simulink model "soc_WLAN_fpga"  (R2024b)
settings: Solver=FixedStepDiscrete  StartTime=0.0  StopTime=stopTime  RelTol=1e-3
PreLoadFcn:
  | addpath(fullfile(matlabroot,'toolbox','whdl','whdlexamples','whdlexamples'));
InitFcn:
  | addpath(fullfile(matlabroot,'toolbox','whdl','whdlexamples','whdlexamples'));
model workspace (MAT data in the model file):
  socvcb : containers.Map (value not decoded)
undefined symbols (not defined in the file): Add, bitRatePerOfdmSym, chanBW, coe, cpLen, dataUpsampleFactor, DelayValMaxNsdMinusLastPilotSc, DescramblerInitialSeed, designMultirateFIR, fftLen, filterLatency, filterUpsampleFactor, Fs, Hd, HT_MFMCS0, HT_MFMCS1, HT_MFMCS2, HT_MFMCS3, HT_MFMCS4, HT_MFMCS5, HT_MFMCS6, HT_MFMCS7, HTUnUsedScInd, inputSamplingRate, interp_coeff, maxPilotRefCounterVale, maxPilotsRef, maxPilotsRefNonHT, Ncol_HT, Ncol_NonHT, noDataSubCarriers, Non_HTMCS0, Non_HTMCS1, Non_HTMCS2, Non_HTMCS3, Non_HTMCS4, Non_HTMCS5, Non_HTMCS6, Non_HTMCS7, Nrow_HT, Nrow_NonHT, numDSC_HT, numDSC_HT_vhtSigB, numDSC_NonHT, numDscHT, numDscNonHT, numOfBitsPerOFDMSym, numOfDataBitsPerOFDMSym, numPilots, numScHT, numSCS_HT, numSCS_NonHT, pnSeq, QAM, rxDownsampleFactor, secondPIdx_HT, secondPIdx_NonHT, Shift, VHTMCS0, VHTMCS1 ... (+7)
libraries: hdlsllib x267, simulink x210, dspsigops x22, whdlutilities x10, whdlmod x9, dsphdlfiltering2 x5, dsphdlmathfun2 x4, whdledac x3, hwlogicconnlib x2, commhdlcrc x2, dsphdlsigops2 x2
(part 4 of 14)

== system soc_WLAN_fpga/WLAN/WLAN HDL/WLAN_Tx_Rx/WLAN_Rx/WLANHDLReceiver/HT_VHTChannelEstAndEqualize/ChannelEqualizer ==
  note: Delay by 1 OFDM Symbol time
  dataIn : Inport
  validIn : Inport  Port=2
  chanEst : Inport  Port=3
  chanEstVal : Inport  Port=4
  chanEstLen : Inport  Port=5
  syncStart : Inport  Port=6
  symbNum : Inport  Port=7
  Delay1 : Delay  DelayLength=1
  Delay11 : Delay  DelayLength=1
  Delay2 : Delay  DelayLength=1
  Delay3 : Delay  DelayLength=80
  Delay4 : Delay  DelayLength=80
  Delay{5..6,8..9} (4 alike) : Delay
  HDL Counter : hdlsllib/Sources/HDL Counter  CountType=Count limited  CountInit=0  CountStep=1  CountMax=numSCS_HT-1  CountFromType=Initial value  CountFrom=0  CountResetPort=on  CountLoadPort=off  CountEnbPort=on  CountDirPort=off  CountHitOutputPort=off  CountDataType=Unsigned  CountWordLen=8  CountFracLen=0  CountSampTime=1
  HDL Counter1 : hdlsllib/Sources/HDL Counter  CountType=Count limited  CountInit=0  CountStep=1  CountMax=numSCS_HT-1  CountFromType=Initial value  CountFrom=0  CountResetPort=on  CountLoadPort=off  CountEnbPort=on  CountDirPort=off  CountHitOutputPort=off  CountDataType=Unsigned  CountWordLen=8  CountFracLen=0  CountSampTime=1
  OFDM Equalizer : whdlmod/OFDM Equalizer  EqualizationMethod=ZF  MaxLenChEstiPerSym=numSCS_HT  resetPort=on
  Simple Dual Port RAM1 : hdlsllib/HDL RAMs/Simple Dual Port RAM  ram_size=8
  validForEqualization : Subsystem
  dataOut : Outport
  validOut : Outport  Port=2
  wires:
  validForEqualization/1(hValid) -> HDL Counter1/2
  HDL Counter/1 -> Simple Dual Port RAM1/2
  validIn/1 -> validForEqualization/1(validIn)
  Delay11/1 -> Simple Dual Port RAM1/4
  HDL Counter1/1 -> Delay11/1
  Delay9/1 -> OFDM Equalizer/1
  Delay3/1 -> Delay1/1
  Delay8/1 -> OFDM Equalizer/4
  Delay6/1 -> OFDM Equalizer/5
  validForEqualization/3(loadH) -> Delay6/1
  Simple Dual Port RAM1/1 -> OFDM Equalizer/2
  Delay5/1 -> OFDM Equalizer/3
  dataIn/1 -> Delay9/1
  symbNum/1 -> validForEqualization/2(symbNum)
  Delay4/1 -> Delay2/1
  chanEstVal/1 -> Delay4/1
  chanEstLen/1 -> Delay8/1
  validForEqualization/2(DataValid) -> Delay5/1
  chanEst/1 -> Delay3/1
  OFDM Equalizer/2 -> validOut/1
  OFDM Equalizer/1 -> dataOut/1
  syncStart/1 -> HDL Counter1/1, validForEqualization/3(rst), OFDM Equalizer/6, HDL Counter/1
  Delay1/1 -> Simple Dual Port RAM1/1
  Delay2/1 -> Simple Dual Port RAM1/3, HDL Counter/2

== system soc_WLAN_fpga/WLAN/WLAN HDL/WLAN_Tx_Rx/WLAN_Rx/WLANHDLReceiver/HT_VHTChannelEstAndEqualize/ChannelEstimator ==
  note: Selecting 9th symbol i.e., HT/VHT LTF after OFDM demod
  note: Sending chan est as 1 when valid is low to channel equalizer
  dataIn : Inport
  validIn : Inport  Port=2
  syncStart : Inport  Port=3
  symbNum : Inport  Port=4
  1-D Lookup Table1 : Lookup_n-D  NumberOfTableDimensions=1  BreakpointsForDimension1=0:length(wlanConfig.fdhtltf)-1  IndexSearchMethod=Evenly spaced points  Table=[wlanConfig.fdhtltf]  TableDataTypeStr=fixdt(1,2,0)  ExtrapMethod=Clip  UseLastTableValue=on  InternalRulePriority=Speed  OutDataTypeStr=fixdt(1,2,0)  RndMeth=Simplest
  Compare To Constant2 : simulink/Logic and Bit Operations/Compare To Constant  relop===  const=8  OutDataTypeStr=boolean
  Constant1 : Constant  Value=numSCS_HT  OutDataTypeStr=fixdt(0,16,0)  SampleTime=-1
  Constant2 : Constant  Value=complex(1,0)  OutDataTypeStr=fixdt(1,16,14)  SampleTime=-1
  Delay{,1..3} (4 alike) : Delay  DelayLength=1  InitialCondition=0  UseCircularBuffer=on
  HDL Counter1 : hdlsllib/Sources/HDL Counter  CountType=Count limited  CountInit=0  CountStep=1  CountMax=numSCS_HT-1  CountFromType=Initial value  CountFrom=0  CountResetPort=on  CountLoadPort=off  CountEnbPort=on  CountDirPort=off  CountHitOutputPort=off  CountDataType=Unsigned  CountWordLen=16  CountFracLen=0  CountSampTime=1
  Logical Operator1 : Logic  AllPortsSameDT=off  OutDataTypeStr=boolean
  OFDM Channel Estimator : whdlmod/OFDM Channel Estimator  timeAvgCheckBox=off  numOFDMSymToBeAvg=2  enableInterpCheckBox=off  interpFac=3  maxNumSubCarPerSym=52  resetPort=on
  Switch : Switch  Criteria=u2 > Threshold  SaturateOnIntegerOverflow=off  InputSameDT=off
  HT_VHTchanEst : Outport
  HT_VHTchanEstValid : Outport  Port=2
  chanEstLen : Outport  Port=3
  wires:
  HDL Counter1/1 -> 1-D Lookup Table1/1
  Compare To Constant2/1 -> Logical Operator1/2
  Constant1/1 -> chanEstLen/1
  syncStart/1 -> OFDM Channel Estimator/5, HDL Counter1/1
  validIn/1 -> Logical Operator1/1
  symbNum/1 -> Compare To Constant2/1
  Switch/1 -> HT_VHTchanEst/1
  OFDM Channel Estimator/1 -> Switch/1
  OFDM Channel Estimator/2 -> Switch/2, HT_VHTchanEstValid/1
  Constant2/1 -> Switch/3
  1-D Lookup Table1/1 -> Delay/1
  dataIn/1 -> Delay1/1
  Delay/1 -> OFDM Channel Estimator/3
  Delay1/1 -> OFDM Channel Estimator/1
  Logical Operator1/1 -> Delay2/1, Delay3/1, HDL Counter1/2
  Delay2/1 -> OFDM Channel Estimator/4
  Delay3/1 -> OFDM Channel Estimator/2

== system soc_WLAN_fpga/WLAN/WLAN HDL/WLAN_Tx_Rx/WLAN_Rx/WLANHDLReceiver/HT_VHTChannelEstAndEqualize/HTScSelector ==
  validIn : Inport
  symbRst : Inport  Port=2
  rst : Inport  Port=3
  1-D Lookup Table : Lookup_n-D  NumberOfTableDimensions=1  BreakpointsForDimension1=[0:length(HTUnUsedScInd)-1]  IndexSearchMethod=Evenly spaced points  Table=HTUnUsedScInd-1  ExtrapMethod=Clip  UseLastTableValue=on  InternalRulePriority=Speed  OutDataTypeStr=uint16  RndMeth=Simplest
  HDL Counter : hdlsllib/Sources/HDL Counter  CountType=Count limited  CountInit=0  CountStep=1  CountMax=length(HTUnUsedScInd)-1  CountFromType=Initial value  CountFrom=0  CountResetPort=on  CountLoadPort=off  CountEnbPort=on  CountDirPort=off  CountHitOutputPort=off  CountDataType=Unsigned  CountWordLen=8  CountFracLen=0  CountSampTime=1
  HDL Counter1 : hdlsllib/Sources/HDL Counter  CountType=Count limited  CountInit=0  CountStep=1  CountMax=fftLen-1  CountFromType=Initial value  CountFrom=0  CountResetPort=on  CountLoadPort=off  CountEnbPort=on  CountDirPort=off  CountHitOutputPort=off  CountDataType=Unsigned  CountWordLen=8  CountFracLen=0  CountSampTime=1
  Logical Operator : Logic  AllPortsSameDT=off  OutDataTypeStr=boolean
  Logical Operator1 : Logic  Operator=OR  AllPortsSameDT=off  OutDataTypeStr=boolean
  Logical Operator2 : Logic  Operator=NOT  AllPortsSameDT=off  OutDataTypeStr=boolean
  Logical Operator3 : Logic  AllPortsSameDT=off  OutDataTypeStr=boolean
  Relational Operator : RelationalOperator  Operator===  OutDataTypeStr=boolean  RndMeth=Simplest  InputSameDT=off
  chanEstValid : Outport
  wires:
  Logical Operator3/1 -> chanEstValid/1
  HDL Counter/1 -> 1-D Lookup Table/1
  Logical Operator2/1 -> Logical Operator3/1
  rst/1 -> Logical Operator1/2
  symbRst/1 -> Logical Operator1/1
  Logical Operator/1 -> HDL Counter/2
  Logical Operator1/1 -> HDL Counter/1, HDL Counter1/1
  1-D Lookup Table/1 -> Relational Operator/1
  Relational Operator/1 -> Logical Operator/2, Logical Operator2/1
  validIn/1 -> Logical Operator3/2, HDL Counter1/2, Logical Operator/1
  HDL Counter1/1 -> Relational Operator/2

== system soc_WLAN_fpga/WLAN/WLAN HDL/WLAN_Tx_Rx/WLAN_Rx/WLANHDLReceiver/HT_VHTChannelEstAndEqualize/ValidController ==
  note: Select VHTSigB symbol for frame format 2
  note: Selecting only VHT data for frame format 2
  symbNum : Inport
  formatDetected : Inport  Port=2
  validIn : Inport  Port=3
  Compare To Constant : simulink/Logic and Bit Operations/Compare To Constant  relop===  const=9  OutDataTypeStr=boolean
  Compare To Constant1 : simulink/Logic and Bit Operations/Compare To Constant  relop===  const=2  OutDataTypeStr=boolean
  Logical Operator : Logic  AllPortsSameDT=off  OutDataTypeStr=boolean
  Logical Operator1 : Logic  Operator=NOT  AllPortsSameDT=off  OutDataTypeStr=boolean
  Logical Operator2 : Logic  AllPortsSameDT=off  OutDataTypeStr=boolean
  Logical Operator4 : Logic  AllPortsSameDT=off  OutDataTypeStr=boolean
  validOut : Outport
  vhtSigB : Outport  Port=2
  wires:
  Logical Operator1/1 -> Logical Operator2/1
  Compare To Constant1/1 -> Logical Operator/1
  symbNum/1 -> Compare To Constant/1
  Compare To Constant/1 -> Logical Operator/2
  Logical Operator2/1 -> validOut/1
  validIn/1 -> Logical Operator2/2, Logical Operator4/2
  formatDetected/1 -> Compare To Constant1/1
  Logical Operator4/1 -> vhtSigB/1
  Logical Operator/1 -> Logical Operator4/1, Logical Operator1/1

== system soc_WLAN_fpga/WLAN/WLAN HDL/WLAN_Tx_Rx/WLAN_Rx/WLANHDLReceiver/NonHTCPEEstAndCorrection/CPECorrector ==
  note: Let Z be the complex CPE estimate and Xbar be the data and X be the corrected data.
      |
      | X = Xbar * conj(Z) * (1/abs(Z))
  dataIn : Inport
  validIn : Inport  Port=2
  estimate : Inport  Port=3
  Complex to Magnitude-Angle HDL Optimized : dsphdlmathfun2/Complex to Magnitude-Angle  NumIterationsSource=Auto  NumIterations=10  OutputFormat=Magnitude  AngleFormat=Normalized  ScaleOutput=on  ScalingMethod=Shift-Add  SimulateUsing=Code generation
  Constant1 : Constant  OutMin=1  OutMax=1  OutDataTypeStr=boolean  SampleTime=1/Fs
  Data Type Conversion : DataTypeConversion  OutDataTypeStr=fixdt(1,16,10)  SaturateOnIntegerOverflow=off  RndMeth=Floor
  Data Type Conversion1 : DataTypeConversion  OutDataTypeStr=fixdt(1,16,14)  SaturateOnIntegerOverflow=off  RndMeth=Floor
  Data Type Conversion : DataTypeConversion  OutDataTypeStr=fixdt(1,14,9)  SaturateOnIntegerOverflow=off  RndMeth=Floor
  Delay : Delay  DelayLength=20
  Delay1 : Delay  DelayLength=20
  Delay{2..4,6..8,10,14..18,22,25,28,36,39} (17 alike) : Delay  InitialCondition=0
  Delay11 : Delay  DelayLength=7  InitialCondition=0
  Delay12 : Delay  DelayLength=7  InitialCondition=0
  Delay5 : Delay  DelayLength=20
  Delay9 : Delay  DelayLength=7  InitialCondition=0
  Math Function : Math  Operator=conj  SignedPower=on  RndMeth=Zero
  Product1 : Product  OutDataTypeStr=Inherit: Same as first input
  Product2 : Product  OutDataTypeStr=Inherit: Same as first input
  Reciprocal : Subsystem  mask{WL=14, FL=9, outWL=26, Mapp=RAM - Based}
      mask prompts: WL "Input Word Length :"; FL "Input Fractional Length :"; outWL "Output Word Length :"; Mapp "Mapping Type:"
      mask init: same as soc_WLAN_fpga/WLAN/WLAN HDL/WLAN_Tx_Rx/WLAN_Rx/WLANHDLReceiver/HT_VHTCPEEstAndCorrection/CPECorrector/Reciprocal
      mask TypeOptions Mapp: LUT - Based | RAM - Based
      mask DialogControl DescGroupVar Prompt: LUT - Based function
      mask DialogControl DescTextVar Prompt: This block is implemented for complex reciprocal
      mask Display: disp(['Reciprocal\n' get_param(gcb,'Mapp') '\nLatency = 7'])
  Terminator : Terminator
  dataOut : Outport
  validOut : Outport  Port=2
  wires:
  Delay7/1 -> Delay17/1
  Complex to Magnitude-Angle HDL Optimized/1 -> Delay10/1
  Constant1/1 -> Complex to Magnitude-Angle HDL Optimized/2
  Product1/1 -> Delay39/1
  estimate/1 -> Complex to Magnitude-Angle HDL Optimized/1, Delay1/1
  Delay36/1 -> Product2/1
  Delay1/1 -> Delay25/1
  Delay25/1 -> Delay9/1
  Math Function/1 -> Delay28/1
  Delay28/1 -> Product2/2
  Delay16/1 -> Delay18/1
  Delay22/1 -> validOut/1
  Delay39/1 -> Data Type Conversion1/1
  Product2/1 -> Delay4/1
  Delay14/1 -> Delay16/1
  Delay2/1 -> Delay12/1
  Delay5/1 -> Delay2/1
  validIn/1 -> Delay5/1
  dataIn/1 -> Data Type Conversion/1
  Delay/1 -> Delay8/1
  Delay8/1 -> Delay11/1
  Delay4/1 -> Delay15/1
  Delay6/1 -> Terminator/1
  Delay9/1 -> Math Function/1
  Delay11/1 -> Delay36/1
  Delay12/1 -> Delay14/1
  Delay15/1 -> Product1/1
  Delay17/1 -> Product1/2
  Delay18/1 -> Delay22/1
  Delay3/1 -> Delay7/1
  Delay10/1 -> Data Type Conversion/1
  Complex to Magnitude-Angle HDL Optimized/2 -> Delay6/1
  Data Type Conversion/1 -> Reciprocal/1(dataIn)
  Data Type Conversion/1 -> Delay/1
  Data Type Conversion1/1 -> dataOut/1
  Reciprocal/1(dataOut) -> Delay3/1

== system soc_WLAN_fpga/WLAN/WLAN HDL/WLAN_Tx_Rx/WLAN_Rx/WLANHDLReceiver/NonHTCPEEstAndCorrection/CPEEstimator ==
  note: delay the adder output till the end of Symbol
      | delay value = Maximum Used subcarrier-
      |  Last pilot Subcarrier position
  note: add the pilots; reset the pilots for every Symbol
  note: Multiply the Equalizer Output with reference pilots
  dataOut : Inport
  pilotScValid : Inport  Port=2
  SymbolEndInd : Inport  Port=3
  polarity : Inport  Port=4
  rst : Inport  Port=5
  Add : Sum  OutDataTypeStr=Inherit: Same as first input
  Constant : Constant  Value=complex(0,0)  OutDataTypeStr=Inherit: Inherit via back propagation  SampleTime=-1
  Constant1 : Constant  Value=0  OutDataTypeStr=Inherit: Inherit via back propagation  SampleTime=-1
  Data Type Conversion : DataTypeConversion  OutDataTypeStr=fixdt(1,16,8)  SaturateOnIntegerOverflow=off  RndMeth=Floor
  Delay : Delay  DelayLength=1  ExternalReset=Level
      settings: InputPortMap=u0,r5
  Delay1 : Delay  DelayLength=DelayValMaxNsdMinusLastPilotSc
  Delay{2..5} (4 alike) : Delay  DelayLength=1  InitialCondition=0  UseCircularBuffer=on
  Product : Product  OutDataTypeStr=Inherit: Same as first input
  Product1 : Product  OutDataTypeStr=Inherit: Same as first input
  Real-Imag to Complex : RealImagToComplex
  RefrenceSignalGen : Subsystem
  Switch : Switch  Criteria=u2 > Threshold  SaturateOnIntegerOverflow=off  InputSameDT=off
  sampleAndHold : MATLAB Function  TreatAsAtomicUnit=on
  x : Outport
  wires:
  Delay1/1 -> sampleAndHold/1(x)
  Switch/1 -> Add/1
  Constant/1 -> Switch/3
  pilotScValid/1 -> Delay4/1, RefrenceSignalGen/1(loadIn)
  dataOut/1 -> Delay5/1
  Constant1/1 -> Real-Imag to Complex/2
  Delay/1 -> Add/2
  Real-Imag to Complex/1 -> Product1/1
  Add/1 -> Delay1/1, Delay/1
  Product/1 -> Data Type Conversion/1
  RefrenceSignalGen/1(RefPilotsOut) -> Real-Imag to Complex/1
  SymbolEndInd/1 -> Delay/2, sampleAndHold/2(enb)
  Product1/1 -> Product/2
  polarity/1 -> Delay3/1
  rst/1 -> sampleAndHold/3(rst), RefrenceSignalGen/2(rst)
  Data Type Conversion/1 -> Switch/1
  sampleAndHold/1(y) -> Delay2/1
  Delay2/1 -> x/1
  Delay3/1 -> Product1/2
  Delay4/1 -> Switch/2
  Delay5/1 -> Product/1

== system soc_WLAN_fpga/WLAN/WLAN HDL/WLAN_Tx_Rx/WLAN_Rx/WLANHDLReceiver/NonHTCPEEstAndCorrection/DataSubCarrierSelector ==
  note: Pilot Subcarriers are stored in LUT. Note that subcarriers positions other than pilots subcarriers positions are stored with Max Value outside the range of Subcarriers (65 for 20Mhz)
  note: Count Used Subcarriers and generate pulse at the end of the Symbol
  note: Pilot Subcarriers are selected by comparing with counter value and LUT output
  EqValidIn : Inport
  rst : Inport  Port=2
  1-D Lookup Table : Lookup_n-D  NumberOfTableDimensions=1  BreakpointsForDimension1=[0:numSCS_NonHT-1]  IndexSearchMethod=Evenly spaced points  Table=NonHTLUTPilots.'  TableDataTypeStr=uint8  ExtrapMethod=Clip  UseLastTableValue=on  InternalRulePriority=Speed  OutDataTypeStr=uint8  RndMeth=Simplest
  Delay1 : Delay  DelayLength=1  InitialCondition=0  UseCircularBuffer=on
  Delay15 : Delay  DelayLength=1  InitialCondition=0  UseCircularBuffer=on
  Delay2 : Delay  DelayLength=1  InitialCondition=0  UseCircularBuffer=on
  HDL Counter : hdlsllib/Sources/HDL Counter  CountType=Count limited  CountInit=0  CountStep=1  CountMax=numSCS_NonHT-1  CountFromType=Initial value  CountFrom=0  CountResetPort=on  CountLoadPort=off  CountEnbPort=on  CountDirPort=off  CountHitOutputPort=on  CountDataType=Unsigned  CountWordLen=maxNsdCounterWL  CountFracLen=0  CountSampTime=1
  Logical Operator : Logic  Operator=NOT  AllPortsSameDT=off  OutDataTypeStr=boolean
  Logical Operator1 : Logic  AllPortsSameDT=off  OutDataTypeStr=boolean
  Relational Operator : RelationalOperator  Operator===  OutDataTypeStr=boolean  RndMeth=Simplest  InputSameDT=off
  Terminator : Terminator
  dataScValidOut : Outport  VectorParamsAs1DForOutWhenUnconnected=off
  wires:
  EqValidIn/1 -> Delay2/1, HDL Counter/2
  HDL Counter/1 -> 1-D Lookup Table/1, Delay1/1
  1-D Lookup Table/1 -> Delay15/1
  Relational Operator/1 -> Logical Operator/1
  HDL Counter/2 -> Terminator/1
  Logical Operator/1 -> Logical Operator1/2
  Logical Operator1/1 -> dataScValidOut/1
  rst/1 -> HDL Counter/1
  Delay15/1 -> Relational Operator/1
  Delay1/1 -> Relational Operator/2
  Delay2/1 -> Logical Operator1/1

== system soc_WLAN_fpga/WLAN/WLAN HDL/WLAN_Tx_Rx/WLAN_Rx/WLANHDLReceiver/NonHTCPEEstAndCorrection/PilotSubCarrierSelector ==
  note: Pilot Subcarriers are stored in LUT. Note that subcarriers positions other than pilots subcarriers positions are stored with Max Value outside the range of Subcarriers
  note: Count Used Subcarriers and generate pulse at the end of the Symbol
  note: Pilot Subcarriers are selected by comparing with counter value and LUT output
  EqValidIn : Inport
  rst : Inport  Port=2
  1-D Lookup Table : Lookup_n-D  NumberOfTableDimensions=1  BreakpointsForDimension1=[0:numSCS_NonHT-1]  IndexSearchMethod=Evenly spaced points  Table=NonHTLUTPilots.'  ExtrapMethod=Clip  UseLastTableValue=on  InternalRulePriority=Speed  OutDataTypeStr=uint8  RndMeth=Simplest
  Compare To Zero : simulink/Logic and Bit Operations/Compare To Zero  relop===  OutDataTypeStr=boolean
  Delay{1..4,15} (5 alike) : Delay  DelayLength=1  InitialCondition=0  UseCircularBuffer=on
  HDL Counter : hdlsllib/Sources/HDL Counter  CountType=Count limited  CountInit=0  CountStep=1  CountMax=numSCS_NonHT-1  CountFromType=Initial value  CountFrom=0  CountResetPort=on  CountLoadPort=off  CountEnbPort=on  CountDirPort=off  CountHitOutputPort=on  CountDataType=Unsigned  CountWordLen=maxNsdCounterWL  CountFracLen=0  CountSampTime=1
  Logical Operator : Logic  AllPortsSameDT=off  OutDataTypeStr=boolean
  Relational Operator : RelationalOperator  Operator===  OutDataTypeStr=boolean  RndMeth=Simplest  InputSameDT=off
  pilotScValidOut : Outport  VectorParamsAs1DForOutWhenUnconnected=off
  SymbEndInd : Outport  Port=2  VectorParamsAs1DForOutWhenUnconnected=off
  SymbStart : Outport  Port=3  VectorParamsAs1DForOutWhenUnconnected=off
  wires:
  EqValidIn/1 -> Delay4/1, HDL Counter/2
  HDL Counter/1 -> Delay1/1, Delay3/1, 1-D Lookup Table/1
  1-D Lookup Table/1 -> Delay15/1
  Relational Operator/1 -> pilotScValidOut/1
  HDL Counter/2 -> Delay2/1
  Compare To Zero/1 -> Logical Operator/1
  Logical Operator/1 -> SymbStart/1
  rst/1 -> HDL Counter/1
  Delay15/1 -> Relational Operator/1
  Delay1/1 -> Relational Operator/2
  Delay2/1 -> SymbEndInd/1
  Delay3/1 -> Compare To Zero/1
  Delay4/1 -> Logical Operator/2

== system soc_WLAN_fpga/WLAN/WLAN HDL/WLAN_Tx_Rx/WLAN_Rx/WLANHDLReceiver/NonHTCPEEstAndCorrection/PolarityGenerator ==
  note: Choose polarity 1 for L-SIG
  enb : Inport
  rstIn : Inport  Port=2
  1-D Lookup Table : Lookup_n-D  NumberOfTableDimensions=1  BreakpointsForDimension1=0:126  BreakpointsForDimension1FirstPoint=0  IndexSearchMethod=Evenly spaced points  Table=pnSeq  TableDataTypeStr=fixdt(1,2,0)  ExtrapMethod=Clip  UseLastTableValue=on  InternalRulePriority=Speed  OutDataTypeStr=fixdt(1,2,0)  RndMeth=Simplest
  Compare To Zero : simulink/Logic and Bit Operations/Compare To Zero  relop===  OutDataTypeStr=boolean
  Constant : Constant  Value=fi(1,1,2,0)  SampleTime=-1
  Delay1 : Delay  DelayLength=1  InitialCondition=0  UseCircularBuffer=on
  Delay2 : Delay  DelayLength=1  InitialCondition=0  UseCircularBuffer=on
  HDL Counter : hdlsllib/Sources/HDL Counter  CountType=Count limited  CountInit=0  CountStep=1  CountMax=126  CountFromType=Initial value  CountFrom=0  CountResetPort=on  CountLoadPort=off  CountEnbPort=on  CountDirPort=off  CountHitOutputPort=off  CountDataType=Unsigned  CountWordLen=7  CountFracLen=0  CountSampTime=1
  HDL Counter1 : hdlsllib/Sources/HDL Counter  CountType=Count limited  CountInit=0  CountStep=1  CountMax=65535  CountFromType=Initial value  CountFrom=0  CountResetPort=on  CountLoadPort=off  CountEnbPort=on  CountDirPort=off  CountHitOutputPort=off  CountDataType=Unsigned  CountWordLen=16  CountFracLen=0  CountSampTime=1
  Logical Operator : Logic  AllPortsSameDT=off  OutDataTypeStr=boolean
  Logical Operator1 : Logic  Operator=OR  AllPortsSameDT=off  OutDataTypeStr=boolean
  Switch : Switch  Criteria=u2 ~= 0  SaturateOnIntegerOverflow=off  InputSameDT=off
  polarity : Outport
  wires:
  enb/1 -> Logical Operator/2, HDL Counter1/2, HDL Counter/2
  HDL Counter/1 -> 1-D Lookup Table/1
  HDL Counter1/1 -> Compare To Zero/1
  Compare To Zero/1 -> Logical Operator/1
  Logical Operator/1 -> Logical Operator1/2, Delay1/1
  Constant/1 -> Switch/1
  1-D Lookup Table/1 -> Delay2/1
  Switch/1 -> polarity/1
  rstIn/1 -> Logical Operator1/1, HDL Counter1/1
  Logical Operator1/1 -> HDL Counter/1
  Delay2/1 -> Switch/3
  Delay1/1 -> Switch/2

== system soc_WLAN_fpga/WLAN/WLAN HDL/WLAN_Tx_Rx/WLAN_Rx/WLANHDLReceiver/NonHTChannelEstAndEqualize/ChannelEqualizer ==
  note: Delay by 1 OFDM Symbol time
  dataIn : Inport
  validIn : Inport  Port=2
  chanEst : Inport  Port=3
  chanEstVal : Inport  Port=4
  chanEstLen : Inport  Port=5
  symbNum : Inport  Port=6
  rst : Inport  Port=7
  Compare To Zero : simulink/Logic and Bit Operations/Compare To Zero  relop===  OutDataTypeStr=boolean
  Delay3 : Delay  DelayLength=fftLen+cpLen
  Delay4 : Delay  DelayLength=fftLen+cpLen
  HDL Counter : hdlsllib/Sources/HDL Counter  CountType=Count limited  CountInit=0  CountStep=1  CountMax=numSCS_NonHT-1  CountFromType=Initial value  CountFrom=0  CountResetPort=on  CountLoadPort=off  CountEnbPort=on  CountDirPort=off  CountHitOutputPort=off  CountDataType=Unsigned  CountWordLen=8  CountFracLen=0  CountSampTime=1
  Logical Operator : Logic  AllPortsSameDT=off  OutDataTypeStr=boolean
  NonHTDataSelector : Subsystem
  OFDM Equalizer : whdlmod/OFDM Equalizer  EqualizationMethod=ZF  MaxLenChEstiPerSym=numSCS_NonHT  resetPort=on
  dataOut : Outport
  validOut : Outport  Port=2
  wires:
  dataIn/1 -> OFDM Equalizer/1
  validIn/1 -> NonHTDataSelector/1(validIn)
  OFDM Equalizer/1 -> dataOut/1
  OFDM Equalizer/2 -> validOut/1
  chanEstVal/1 -> Delay3/1
  chanEst/1 -> Delay4/1
  chanEstLen/1 -> OFDM Equalizer/4
  NonHTDataSelector/1(NonHTValid) -> OFDM Equalizer/3
  HDL Counter/1 -> Compare To Zero/1
  Logical Operator/1 -> OFDM Equalizer/5
  Compare To Zero/1 -> Logical Operator/1
  Delay4/1 -> OFDM Equalizer/2
  Delay3/1 -> Logical Operator/2, HDL Counter/2
  symbNum/1 -> NonHTDataSelector/2(symbNum)
  rst/1 -> OFDM Equalizer/6, HDL Counter/1

== system soc_WLAN_fpga/WLAN/WLAN HDL/WLAN_Tx_Rx/WLAN_Rx/WLANHDLReceiver/NonHTChannelEstAndEqualize/ChannelEstimator ==
  note: Sending chan est as 1 when valid is low to channel equalizer
  note: Selecting LLTF 1 and 2 for channel estimation
  dataIn : Inport
  validIn : Inport  Port=2
  symbNum : Inport  Port=3
  syncStart : Inport  Port=4
  1-D Lookup Table : Lookup_n-D  NumberOfTableDimensions=1  BreakpointsForDimension1=0:length([wlanConfig.fdlltf])-1  IndexSearchMethod=Evenly spaced points  Table=[wlanConfig.fdlltf]  TableDataTypeStr=fixdt(1,2,0)  ExtrapMethod=Clip  UseLastTableValue=on  InternalRulePriority=Speed  OutDataTypeStr=fixdt(1,2,0)  RndMeth=Simplest
  Compare To Constant3 : simulink/Logic and Bit Operations/Compare To Constant  relop=>=  const=2  OutDataTypeStr=boolean
  Compare To Constant4 : simulink/Logic and Bit Operations/Compare To Constant  relop=<=  const=3  OutDataTypeStr=boolean
  Constant : Constant  Value=numSCS_NonHT  OutDataTypeStr=uint8  SampleTime=-1
  Constant1 : Constant  Value=complex(1,0)  OutDataTypeStr=fixdt(1,16,14)  SampleTime=-1
  Data Type Conversion : DataTypeConversion  OutDataTypeStr=fixdt(1,16,14)  SaturateOnIntegerOverflow=off  RndMeth=Floor
  Delay{1..3,15} (4 alike) : Delay  DelayLength=1  InitialCondition=0  UseCircularBuffer=on
  HDL Counter1 : hdlsllib/Sources/HDL Counter  CountType=Count limited  CountInit=0  CountStep=1  CountMax=numSCS_NonHT - 1  CountFromType=Initial value  CountFrom=0  CountResetPort=on  CountLoadPort=off  CountEnbPort=on  CountDirPort=off  CountHitOutputPort=off  CountDataType=Unsigned  CountWordLen=16  CountFracLen=0  CountSampTime=1
  Logical Operator : Logic  Inputs=3  AllPortsSameDT=off  OutDataTypeStr=boolean
  OFDM Channel Estimator : whdlmod/OFDM Channel Estimator  timeAvgCheckBox=on  numOFDMSymToBeAvg=2  enableInterpCheckBox=off  interpFac=3  maxNumSubCarPerSym=numSCS_NonHT  resetPort=on
  Switch : Switch  Criteria=u2 > Threshold  SaturateOnIntegerOverflow=off  InputSameDT=off
  chanEst : Outport
  chanEstValid : Outport  Port=2
  chanEstLen : Outport  Port=3
  wires:
  HDL Counter1/1 -> 1-D Lookup Table/1
  1-D Lookup Table/1 -> Delay15/1
  OFDM Channel Estimator/2 -> Switch/2, chanEstValid/1
  Constant/1 -> chanEstLen/1, OFDM Channel Estimator/5
  syncStart/1 -> OFDM Channel Estimator/6, HDL Counter1/1
  validIn/1 -> Logical Operator/3
  symbNum/1 -> Compare To Constant3/1, Compare To Constant4/1
  Compare To Constant3/1 -> Logical Operator/1
  Compare To Constant4/1 -> Logical Operator/2
  Logical Operator/1 -> Delay2/1, Delay1/1, HDL Counter1/2
  dataIn/1 -> Data Type Conversion/1
  Constant1/1 -> Switch/3
  Switch/1 -> chanEst/1
  OFDM Channel Estimator/1 -> Switch/1
  Delay15/1 -> OFDM Channel Estimator/3
  Delay1/1 -> OFDM Channel Estimator/4
  Delay2/1 -> OFDM Channel Estimator/2
  Data Type Conversion/1 -> Delay3/1
  Delay3/1 -> OFDM Channel Estimator/1

== system soc_WLAN_fpga/WLAN/WLAN HDL/WLAN_Tx_Rx/WLAN_Rx/WLANHDLReceiver/NonHTChannelEstAndEqualize/NonHTScSelector ==
  validIn : Inport
  symbRst : Inport  Port=2
  rst : Inport  Port=3
  1-D Lookup Table : Lookup_n-D  NumberOfTableDimensions=1  BreakpointsForDimension1=[0:length(noDataSubCarriers)-1]  IndexSearchMethod=Evenly spaced points  Table=noDataSubCarriers-1  ExtrapMethod=Clip  UseLastTableValue=on  InternalRulePriority=Speed  OutDataTypeStr=uint16  RndMeth=Simplest
  HDL Counter : hdlsllib/Sources/HDL Counter  CountType=Count limited  CountInit=0  CountStep=1  CountMax=length(noDataSubCarriers)-1  CountFromType=Initial value  CountFrom=0  CountResetPort=on  CountLoadPort=off  CountEnbPort=on  CountDirPort=off  CountHitOutputPort=off  CountDataType=Unsigned  CountWordLen=8  CountFracLen=0  CountSampTime=1
  HDL Counter1 : hdlsllib/Sources/HDL Counter  CountType=Count limited  CountInit=0  CountStep=1  CountMax=fftLen-1  CountFromType=Initial value  CountFrom=0  CountResetPort=on  CountLoadPort=off  CountEnbPort=on  CountDirPort=off  CountHitOutputPort=off  CountDataType=Unsigned  CountWordLen=8  CountFracLen=0  CountSampTime=1
  Logical Operator : Logic  AllPortsSameDT=off  OutDataTypeStr=boolean
  Logical Operator1 : Logic  Operator=OR  AllPortsSameDT=off  OutDataTypeStr=boolean
  Logical Operator2 : Logic  Operator=NOT  AllPortsSameDT=off  OutDataTypeStr=boolean
  Logical Operator3 : Logic  AllPortsSameDT=off  OutDataTypeStr=boolean
  Relational Operator : RelationalOperator  Operator===  OutDataTypeStr=boolean  RndMeth=Simplest  InputSameDT=off
  chanEstValid : Outport
  wires:
  Logical Operator3/1 -> chanEstValid/1
  HDL Counter/1 -> 1-D Lookup Table/1
  Logical Operator2/1 -> Logical Operator3/1
  rst/1 -> Logical Operator1/2
  symbRst/1 -> Logical Operator1/1
  Logical Operator/1 -> HDL Counter/2
  Logical Operator1/1 -> HDL Counter/1, HDL Counter1/1
  Relational Operator/1 -> Logical Operator/2, Logical Operator2/1
  1-D Lookup Table/1 -> Relational Operator/1
  validIn/1 -> Logical Operator3/2, HDL Counter1/2, Logical Operator/1
  HDL Counter1/1 -> Relational Operator/2

== system soc_WLAN_fpga/WLAN/WLAN HDL/WLAN_Tx_Rx/WLAN_Rx/WLANHDLReceiver/OFDMDemodulation/Symbol Counter ==
  validIn : Inport
  rst : Inport  Port=2
  dataIn : Inport  Port=3
  Compare To Constant : simulink/Logic and Bit Operations/Compare To Constant  relop===  const=fftLen-1  OutDataTypeStr=boolean
  Compare To Constant1 : simulink/Logic and Bit Operations/Compare To Constant  relop===  const=2  OutDataTypeStr=boolean
  Constant : Constant  Value=chanBW  OutDataTypeStr=fixdt(0,3,0)  SampleTime=-1
  Logical Operator : Logic  AllPortsSameDT=off  OutDataTypeStr=boolean
  Switch : Switch  Criteria=u2 ~= 0  SaturateOnIntegerOverflow=off  InputSameDT=off
  sample counter : hdlsllib/Sources/HDL Counter  CountType=Count limited  CountInit=0  CountStep=1  CountMax=fftLen-1  CountFromType=Initial value  CountFrom=0  CountResetPort=on  CountLoadPort=off  CountEnbPort=on  CountDirPort=off  CountHitOutputPort=off  CountDataType=Unsigned  CountWordLen=8  CountFracLen=0  CountSampTime=1
  symbol counter : hdlsllib/Sources/HDL Counter  CountType=Count limited  CountInit=0  CountStep=1  CountMax=65535  CountFromType=Initial value  CountFrom=0  CountResetPort=on  CountLoadPort=off  CountEnbPort=on  CountDirPort=off  CountHitOutputPort=off  CountDataType=Unsigned  CountWordLen=16  CountFracLen=0  CountSampTime=1
  vhtRotation : Subsystem
  count : Outport
  symbolRst : Outport  Port=2
  dataOut : Outport  Port=3
  wires:
  sample counter/1 -> vhtRotation/1(u), Compare To Constant/1
  validIn/1 -> Logical Operator/2, sample counter/2
  symbol counter/1 -> count/1
  Logical Operator/1 -> symbolRst/1, symbol counter/2
  Compare To Constant/1 -> Logical Operator/1
  rst/1 -> symbol counter/1, sample counter/1
  dataIn/1 -> Switch/3, vhtRotation/2(In2)
  vhtRotation/1(dataOut) -> Switch/1
  Constant/1 -> Compare To Constant1/1
  Compare To Constant1/1 -> Switch/2
  Switch/1 -> dataOut/1

== system soc_WLAN_fpga/WLAN/WLAN HDL/WLAN_Tx_Rx/WLAN_Rx/WLANHDLReceiver/WLANTimeAndFrequencySynchronization/Coarse CFO Estimation and Correction ==
  dataIn : Inport
  validIn : Inport  Port=2
  lstfStartIn : Inport  Port=3
  rstIn : Inport  Port=4
  Coarse CFO Correction : Subsystem
  Coarse CFO Estimation : Subsystem
  Freq : Outport
  dataOut : Outport  Port=2
  validOut : Outport  Port=3
  lstfStartOut : Outport  Port=4
  rstOut : Outport  Port=5
  wires:
  Coarse CFO Estimation/3(validData) -> Coarse CFO Correction/3(validIn)
  Coarse CFO Correction/3(validOut) -> validOut/1
  Coarse CFO Estimation/4(lstfStart) -> Coarse CFO Correction/4(lstfStartIn)
  Coarse CFO Estimation/1(Freq) -> Coarse CFO Correction/1(freq)
  lstfStartIn/1 -> Coarse CFO Estimation/3(LSTF_start)
  validIn/1 -> Coarse CFO Estimation/2(validIn)
  Coarse CFO Estimation/5(rstOut) -> Coarse CFO Correction/5(rstIn)
  Coarse CFO Estimation/2(dataOut) -> Coarse CFO Correction/2(dataIn)
  dataIn/1 -> Coarse CFO Estimation/1(dataIn)
  Coarse CFO Correction/2(dataOut) -> dataOut/1
  rstIn/1 -> Coarse CFO Estimation/4(rstIn)
  Coarse CFO Correction/4(lstfStartOut) -> lstfStartOut/1
  Coarse CFO Correction/5(rstOut) -> rstOut/1
  Coarse CFO Correction/1(freqOut) -> Freq/1

== system soc_WLAN_fpga/WLAN/WLAN HDL/WLAN_Tx_Rx/WLAN_Rx/WLANHDLReceiver/WLANTimeAndFrequencySynchronization/Coarse Time Sync ==
  dataIn : Inport
  validIn : Inport  Port=2
  startIn : Inport  Port=3
  Delay4 : Delay  DelayLength=2*wlanConfig.lstfLen+11
  Delay6 : Delay  DelayLength=2*wlanConfig.lstfLen+11
  correlator : Subsystem
  energyCalculator : Subsystem
  peakDetection : Subsystem
  streamSynchrnizer : Subsystem
  dataOut : Outport  VectorParamsAs1DForOutWhenUnconnected=off
  validOut : Outport  Port=2  VectorParamsAs1DForOutWhenUnconnected=off
  lstfStart : Outport  Port=3  VectorParamsAs1DForOutWhenUnconnected=off
  rst : Outport  Port=4  VectorParamsAs1DForOutWhenUnconnected=off
  wires:
  startIn/1 -> rst/1, correlator/3(startIn)
  peakDetection/3(dataOut) -> dataOut/1
  validIn/1 -> correlator/2(validIn), energyCalculator/4(validIn), Delay6/1
  Delay4/1 -> streamSynchrnizer/2(dataIn)
  Delay6/1 -> streamSynchrnizer/3(dataValid)
  correlator/2(validOut) -> energyCalculator/2(corrValidIn), streamSynchrnizer/1(corrValid)
  dataIn/1 -> energyCalculator/3(dataIn), Delay4/1, correlator/1(dataIn)
  peakDetection/2(validOut) -> validOut/1
  energyCalculator/2(energyOut) -> peakDetection/2(energyIn)
  energyCalculator/3(validOut) -> peakDetection/3(corrValid)
  peakDetection/1(lstfStart) -> lstfStart/1
  correlator/1(dataOut) -> energyCalculator/1(corrIn)
  energyCalculator/1(corrOut) -> peakDetection/1(corrIn)
  streamSynchrnizer/1(dataOut) -> peakDetection/4(dataIn)
  streamSynchrnizer/2(validOut) -> peakDetection/5(dataValid)

== system soc_WLAN_fpga/WLAN/WLAN HDL/WLAN_Tx_Rx/WLAN_Rx/WLANHDLReceiver/WLANTimeAndFrequencySynchronization/Fine CFO Estimation and Correction ==
  dataIn : Inport
  validIn : Inport  Port=2
  lstfStartIn : Inport  Port=3
  rstIn : Inport  Port=4
  Fine CFO Correction : Subsystem
  Fine CFO Estimation : Subsystem
  Freq : Outport
  freqValidOut : Outport  Port=2
  dataOut : Outport  Port=3
  validOut : Outport  Port=4
  lstfStartOut : Outport  Port=5
  wires:
  Fine CFO Estimation/4(validOut) -> Fine CFO Correction/4(validIn)
  Fine CFO Estimation/1(Freq) -> Fine CFO Correction/1(freqIn)
  validIn/1 -> Fine CFO Estimation/2(validIn)
  Fine CFO Estimation/5(lstfStart) -> Fine CFO Correction/5(lstfStartIn)
  Fine CFO Estimation/3(dataOut) -> Fine CFO Correction/3(dataIn)
  dataIn/1 -> Fine CFO Estimation/1(dataIn)
  Fine CFO Estimation/2(freqValidOut) -> Fine CFO Correction/2(freqValidIn)
  lstfStartIn/1 -> Fine CFO Estimation/3(LSTF_start)
  rstIn/1 -> Fine CFO Estimation/4(rstIn)
  Fine CFO Correction/5(lstfStartOut) -> lstfStartOut/1
  Fine CFO Correction/4(validOut) -> validOut/1
  Fine CFO Correction/3(dataOut) -> dataOut/1
  Fine CFO Correction/1(freqOut) -> Freq/1
  Fine CFO Correction/2(freqValidOut) -> freqValidOut/1

== system soc_WLAN_fpga/WLAN/WLAN HDL/WLAN_Tx_Rx/WLAN_Rx/WLANHDLReceiver/WLANTimeAndFrequencySynchronization/Fine Time Sync ==
  dataIn : Inport
  validIn : Inport  Port=2
  lstfStartIn : Inport  Port=3
  rstIn : Inport  Port=4
  correlator : Subsystem
  peakSearcher : Subsystem
  dataOut : Outport  VectorParamsAs1DForOutWhenUnconnected=off
  validOut : Outport  Port=2  VectorParamsAs1DForOutWhenUnconnected=off
  lstfStartOut : Outport  Port=3  VectorParamsAs1DForOutWhenUnconnected=off
  rstOut : Outport  Port=4  VectorParamsAs1DForOutWhenUnconnected=off
  wires:
  validIn/1 -> correlator/2(validIn)
  dataIn/1 -> correlator/1(dataIn)
  lstfStartIn/1 -> correlator/3(startIn)
  correlator/1(corrOut) -> peakSearcher/1(corrIn)
  correlator/2(corrValid) -> peakSearcher/2(corrValid)
  correlator/3(startOut) -> peakSearcher/3(startIn)
  peakSearcher/1(lstfStart) -> lstfStartOut/1
  peakSearcher/2(validOut) -> validOut/1
  peakSearcher/3(dataOut) -> dataOut/1
  correlator/4(dataOut) -> peakSearcher/4(dataIn)
  correlator/5(validOut) -> peakSearcher/5(validIn)
  rstIn/1 -> rstOut/1, peakSearcher/6(rstIn), correlator/4(rstIn)

== system soc_WLAN_fpga/WLAN/WLAN HDL/WLAN_Tx_Rx/WLAN_Rx/WLANHDLReceiver/WLANTimeAndFrequencySynchronization/Rx Filter ==
  dataIn : Inport
  validIn : Inport  Port=2
  startIn : Inport  Port=3
  Delay : Delay  DelayLength=33
  Discrete FIR Filter HDL Optimized : dsphdlfiltering2/Discrete FIR Filter  NumeratorSource=Property  Numerator=Hd.Numerator  NumeratorPrototype=[]  FilterStructure=Direct form systolic  SerializationOption=Minimum number of cycles between valid input samples  NumCycles=filterUpsampleFactor  NumberOfMultipliers=2  SimulateUsing=Code generation  roundingMode=Floor  overflowMode=off  CoefficientsDataTypeStr=Inherit: Same word length as input  OutputDataTypeStr=fixdt(1,16,12)  ResetInputPort=on  HDLGlobalReset=off  CoeffMultiplier=Multiplier  UseMultForPow2Coeff=on
  dataOut : Outport
  validOut : Outport  Port=2
  startOut : Outport  Port=3
  wires:
  dataIn/1 -> Discrete FIR Filter HDL Optimized/1
  validIn/1 -> Discrete FIR Filter HDL Optimized/2
  startIn/1 -> Discrete FIR Filter HDL Optimized/3, Delay/1
  Discrete FIR Filter HDL Optimized/2 -> validOut/1
  Delay/1 -> startOut/1
  Discrete FIR Filter HDL Optimized/1 -> dataOut/1

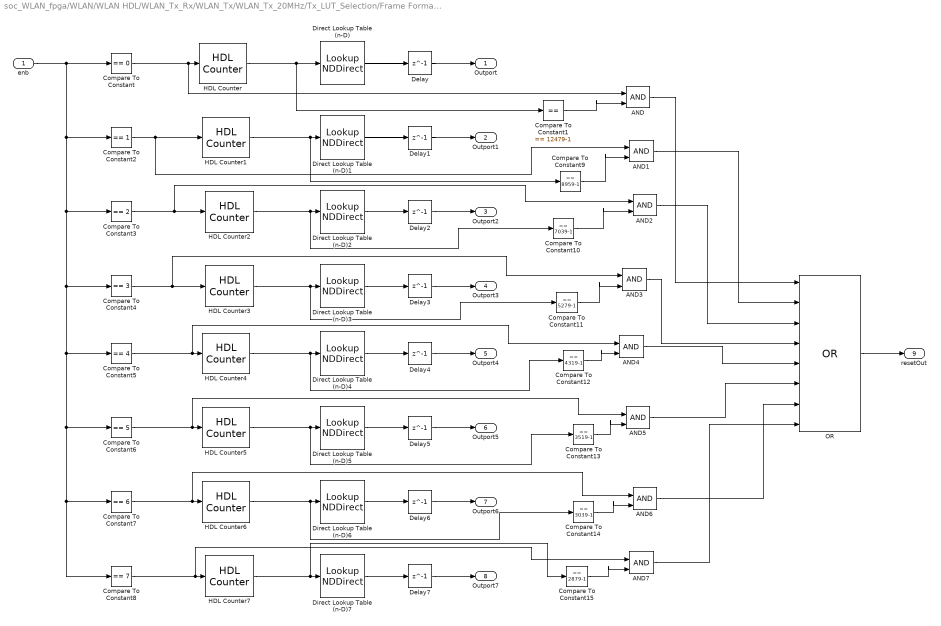
== system soc_WLAN_fpga/WLAN/WLAN HDL/WLAN_Tx_Rx/WLAN_Tx/WLAN_Tx_20MHz/Tx_LUT_Selection/Frame Format 0 ==
  enb : Inport
  AND{,1..7} (8 alike) : Logic  IconShape=distinctive  AllPortsSameDT=off  OutDataTypeStr=boolean
  Compare To Constant : simulink/Logic and Bit Operations/Compare To Constant  relop===  const=0  OutDataTypeStr=boolean
  Compare To Constant1 : simulink/Logic and Bit Operations/Compare To Constant  relop===  const=12479-1  OutDataTypeStr=boolean
  Compare To Constant10 : simulink/Logic and Bit Operations/Compare To Constant  relop===  const=7039-1  OutDataTypeStr=boolean
  Compare To Constant11 : simulink/Logic and Bit Operations/Compare To Constant  relop===  const=5279-1  OutDataTypeStr=boolean
  Compare To Constant12 : simulink/Logic and Bit Operations/Compare To Constant  relop===  const=4319-1  OutDataTypeStr=boolean
  Compare To Constant13 : simulink/Logic and Bit Operations/Compare To Constant  relop===  const=3519-1  OutDataTypeStr=boolean
  Compare To Constant14 : simulink/Logic and Bit Operations/Compare To Constant  relop===  const=3039-1  OutDataTypeStr=boolean
  Compare To Constant15 : simulink/Logic and Bit Operations/Compare To Constant  relop===  const=2879-1  OutDataTypeStr=boolean
  Compare To Constant2 : simulink/Logic and Bit Operations/Compare To Constant  relop===  const=1  OutDataTypeStr=boolean
  Compare To Constant3 : simulink/Logic and Bit Operations/Compare To Constant  relop===  const=2  OutDataTypeStr=boolean
  Compare To Constant4 : simulink/Logic and Bit Operations/Compare To Constant  relop===  const=3  OutDataTypeStr=boolean
  Compare To Constant5 : simulink/Logic and Bit Operations/Compare To Constant  relop===  const=4  OutDataTypeStr=boolean
  Compare To Constant6 : simulink/Logic and Bit Operations/Compare To Constant  relop===  const=5  OutDataTypeStr=boolean
  Compare To Constant7 : simulink/Logic and Bit Operations/Compare To Constant  relop===  const=6  OutDataTypeStr=boolean
  Compare To Constant8 : simulink/Logic and Bit Operations/Compare To Constant  relop===  const=7  OutDataTypeStr=boolean
  Compare To Constant9 : simulink/Logic and Bit Operations/Compare To Constant  relop===  const=8959-1  OutDataTypeStr=boolean
  Delay{,1..7} (8 alike) : Delay  DelayLength=1
  Direct Lookup Table (n-D) : LookupNDDirect  NumberOfTableDimensions=1  Table=Non_HTMCS0
  Direct Lookup Table (n-D)1 : LookupNDDirect  NumberOfTableDimensions=1  Table=Non_HTMCS1
  Direct Lookup Table (n-D)2 : LookupNDDirect  NumberOfTableDimensions=1  Table=Non_HTMCS2
  Direct Lookup Table (n-D)3 : LookupNDDirect  NumberOfTableDimensions=1  Table=Non_HTMCS3
  Direct Lookup Table (n-D)4 : LookupNDDirect  NumberOfTableDimensions=1  Table=Non_HTMCS4
  Direct Lookup Table (n-D)5 : LookupNDDirect  NumberOfTableDimensions=1  Table=Non_HTMCS5
  Direct Lookup Table (n-D)6 : LookupNDDirect  NumberOfTableDimensions=1  Table=Non_HTMCS6
  Direct Lookup Table (n-D)7 : LookupNDDirect  NumberOfTableDimensions=1  Table=Non_HTMCS7
  HDL Counter : hdlsllib/Sources/HDL Counter  CountType=Count limited  CountInit=0  CountStep=1  CountMax=12479  CountFromType=Initial value  CountFrom=0  CountResetPort=off  CountLoadPort=off  CountEnbPort=on  CountDirPort=off  CountHitOutputPort=off  CountDataType=Unsigned  CountWordLen=16  CountFracLen=0  CountSampTime=1
  HDL Counter1 : hdlsllib/Sources/HDL Counter  CountType=Count limited  CountInit=0  CountStep=1  CountMax=8959  CountFromType=Initial value  CountFrom=0  CountResetPort=off  CountLoadPort=off  CountEnbPort=on  CountDirPort=off  CountHitOutputPort=off  CountDataType=Unsigned  CountWordLen=16  CountFracLen=0  CountSampTime=1
  HDL Counter2 : hdlsllib/Sources/HDL Counter  CountType=Count limited  CountInit=0  CountStep=1  CountMax=7039  CountFromType=Initial value  CountFrom=0  CountResetPort=off  CountLoadPort=off  CountEnbPort=on  CountDirPort=off  CountHitOutputPort=off  CountDataType=Unsigned  CountWordLen=16  CountFracLen=0  CountSampTime=1
  HDL Counter3 : hdlsllib/Sources/HDL Counter  CountType=Count limited  CountInit=0  CountStep=1  CountMax=5279  CountFromType=Initial value  CountFrom=0  CountResetPort=off  CountLoadPort=off  CountEnbPort=on  CountDirPort=off  CountHitOutputPort=off  CountDataType=Unsigned  CountWordLen=16  CountFracLen=0  CountSampTime=1
  HDL Counter4 : hdlsllib/Sources/HDL Counter  CountType=Count limited  CountInit=0  CountStep=1  CountMax=4319  CountFromType=Initial value  CountFrom=0  CountResetPort=off  CountLoadPort=off  CountEnbPort=on  CountDirPort=off  CountHitOutputPort=off  CountDataType=Unsigned  CountWordLen=16  CountFracLen=0  CountSampTime=1
  HDL Counter5 : hdlsllib/Sources/HDL Counter  CountType=Count limited  CountInit=0  CountStep=1  CountMax=3519  CountFromType=Initial value  CountFrom=0  CountResetPort=off  CountLoadPort=off  CountEnbPort=on  CountDirPort=off  CountHitOutputPort=off  CountDataType=Unsigned  CountWordLen=16  CountFracLen=0  CountSampTime=1
  HDL Counter6 : hdlsllib/Sources/HDL Counter  CountType=Count limited  CountInit=0  CountStep=1  CountMax=3039  CountFromType=Initial value  CountFrom=0  CountResetPort=off  CountLoadPort=off  CountEnbPort=on  CountDirPort=off  CountHitOutputPort=off  CountDataType=Unsigned  CountWordLen=16  CountFracLen=0  CountSampTime=1
  HDL Counter7 : hdlsllib/Sources/HDL Counter  CountType=Count limited  CountInit=0  CountStep=1  CountMax=2879  CountFromType=Initial value  CountFrom=0  CountResetPort=off  CountLoadPort=off  CountEnbPort=on  CountDirPort=off  CountHitOutputPort=off  CountDataType=Unsigned  CountWordLen=16  CountFracLen=0  CountSampTime=1
  OR : Logic  Operator=OR  Inputs=8  IconShape=distinctive  AllPortsSameDT=off  OutDataTypeStr=boolean
  Outport : Outport
  Outport1 : Outport  Port=2
  Outport2 : Outport  Port=3
  Outport3 : Outport  Port=4
  Outport4 : Outport  Port=5
  Outport5 : Outport  Port=6
  Outport6 : Outport  Port=7
  Outport7 : Outport  Port=8
  resetOut : Outport  Port=9
  wires:
  Direct Lookup Table (n-D)/1 -> Delay/1
  Direct Lookup Table (n-D)1/1 -> Delay1/1
  Direct Lookup Table (n-D)2/1 -> Delay2/1
  Delay/1 -> Outport/1
  Delay1/1 -> Outport1/1
  Delay2/1 -> Outport2/1
  Delay3/1 -> Outport3/1
  Direct Lookup Table (n-D)3/1 -> Delay3/1
  Direct Lookup Table (n-D)5/1 -> Delay5/1
  Direct Lookup Table (n-D)7/1 -> Delay7/1
  Delay4/1 -> Outport4/1
  Direct Lookup Table (n-D)4/1 -> Delay4/1
  Delay7/1 -> Outport7/1
  Delay6/1 -> Outport6/1
  Delay5/1 -> Outport5/1
  Direct Lookup Table (n-D)6/1 -> Delay6/1
  enb/1 -> Compare To Constant/1, Compare To Constant8/1, Compare To Constant7/1, Compare To Constant6/1, Compare To Constant5/1, Compare To Constant4/1, Compare To Constant3/1, Compare To Constant2/1
  Compare To Constant/1 -> AND/1, HDL Counter/1
  HDL Counter/1 -> Direct Lookup Table (n-D)/1, Compare To Constant1/1
  Compare To Constant1/1 -> AND/2
  Compare To Constant2/1 -> AND1/1, HDL Counter1/1
  HDL Counter1/1 -> Compare To Constant9/1, Direct Lookup Table (n-D)1/1
  Compare To Constant3/1 -> HDL Counter2/1, AND2/1
  HDL Counter2/1 -> Compare To Constant10/1, Direct Lookup Table (n-D)2/1
  Compare To Constant4/1 -> HDL Counter3/1, AND3/1
  HDL Counter3/1 -> Compare To Constant11/1, Direct Lookup Table (n-D)3/1
  Compare To Constant5/1 -> AND4/1, HDL Counter4/1
  HDL Counter4/1 -> Compare To Constant12/1, Direct Lookup Table (n-D)4/1
  Compare To Constant6/1 -> AND5/1, HDL Counter5/1
  HDL Counter5/1 -> Compare To Constant13/1, Direct Lookup Table (n-D)5/1
  Compare To Constant7/1 -> AND6/1, HDL Counter6/1
  HDL Counter6/1 -> Compare To Constant14/1, Direct Lookup Table (n-D)6/1
  Compare To Constant8/1 -> AND7/1, HDL Counter7/1
  HDL Counter7/1 -> Compare To Constant15/1, Direct Lookup Table (n-D)7/1
  Compare To Constant9/1 -> AND1/2
  Compare To Constant10/1 -> AND2/2
  Compare To Constant11/1 -> AND3/2
  Compare To Constant12/1 -> AND4/2
  Compare To Constant13/1 -> AND5/2
  Compare To Constant14/1 -> AND6/2
  Compare To Constant15/1 -> AND7/2
  AND/1 -> OR/1
  AND1/1 -> OR/2
  AND2/1 -> OR/3
  AND3/1 -> OR/4
  AND4/1 -> OR/5
  AND5/1 -> OR/6
  AND6/1 -> OR/7
  AND7/1 -> OR/8
  OR/1 -> resetOut/1
